simulink model "simula_PID"  (R2017a)
settings: Solver=VariableStepAuto  StartTime=0.0  StopTime=4000  RelTol=1e-3
values from neighbouring files (symbols this model uses):
  kP = 1.2684    [PI.m]    (also in PID.m = 1; PI_D.m = 1)
  Ti = 1    [PID.m]    (also in PI_D.m)
undefined symbols (not defined in the file or in its folder): Td
libraries: cstblocks x1
settings Model: Creator=Enrico Donato  LastModifiedBy=Enrico Donato

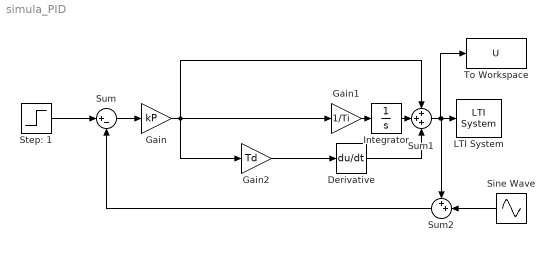
== system simula_PID ==
  Derivative : Derivative
  Gain : Gain  Gain=kP
  Gain1 : Gain  Gain=1/Ti
  Gain2 : Gain  Gain=Td
  Integrator : Integrator
  LTI System : cstblocks/LTI System  sys=G  IC=[]
  Sine Wave : Sin  Amplitude=0.01  Frequency=100  SampleTime=0
  Step: 1 : Step  Time=0  SampleTime=0
  Sum : Sum  Inputs=|+-
  Sum1 : Sum  Inputs=+++
  Sum2 : Sum  Inputs=++|
  To Workspace : ToWorkspace  VariableName=U  SaveFormat=Timeseries  SampleTime=-1
  wires:
  Sum1/1 -> Sum2/1, LTI System/1, To Workspace/1
  Sum/1 -> Gain/1
  Gain1/1 -> Integrator/1
  Integrator/1 -> Sum1/2
  Step: 1/1 -> Sum/1
  Sum2/1 -> Sum/2
  Sine Wave/1 -> Sum2/2
  Gain/1 -> Gain2/1, Sum1/1, Gain1/1
  Derivative/1 -> Sum1/3
  Gain2/1 -> Derivative/1
